simulink model "filter_current"  (R2023b)
settings: Solver=FixedStepDiscrete  StartTime=0.0  StopTime=10.0  FixedStep=FilterCurrent_Ts  RelTol=1e-3  EnableMultiTasking=on
model workspace (MAT data in the model file):
  FilterCurrent_Ts = Simulink.Parameter
  FilterCurrent_Ts.Value = 0.001
  FilterCurrent_Ts.DataType = 'auto'
  FilterCurrent_Ts.DocUnits = 's'
  FilterCurrent_Ts.Complexity = 'real'
  FilterCurrent_Ts.Dimensions = [1 1]
libraries: dspstat3 x1
settings Model: DataDictionary=common.sldd  Creator=ascalzo  LastModifiedBy=mfussi
settings SolverCC: AllowMultiTaskInputOutput=on  AutoInsertRateTranBlk=on  InsertRTBMode=Never (minimum delay)
settings DataIOCC: SaveOutput=off  SignalLogging=off  DSMLogging=off  SaveTime=off  ReturnWorkspaceOutputs=off
settings OptimizationCC: DefaultParameterBehavior=Inlined  UseDivisionForNetSlopeComputation=on  GainParamInheritBuiltInType=on  UseFloatMulNetSlope=on  DefaultUnderspecifiedDataType=single  InlineInvariantSignals=on  PassReuseOutputArgsAs=Individual arguments  ZeroExternalMemoryAtStartup=off  ZeroInternalMemoryAtStartup=off  NoFixptDivByZeroProtection=on  EfficientFloat2IntCast=on  LifeSpan=1  OptimizeBlockOrder=speed  OptimizationPriority=Speed  MultiThreadedLoops=on  EfficientTunableParamExpr=on
settings DebuggingCC: ParameterPrecisionLossMsg=none  UnconnectedInputMsg=warning  UnconnectedOutputMsg=warning  UnconnectedLineMsg=warning
settings HardwareCC: ProdBitPerPointer=32  ProdBitPerSizeT=32  ProdBitPerPtrDiffT=32  ProdLargestAtomicInteger=Long  ProdLargestAtomicFloat=Double  ProdWordSize=32  ProdLongLongMode=on  ProdHWDeviceType=ARM Compatible->ARM Cortex-M
settings ModelReferenceCC: UpdateModelReferenceTargets=Force  EnableRefExpFcnMdlSchedulingChecks=on
settings SFSimCC: MATLABDynamicMemAlloc=off
settings RTWCC: Description=Embedded Coder  SystemTargetFile=ert.tlc  GenCodeOnly=on  PackageGeneratedCodeAndArtifacts=on  PackageName=filter_current  TemplateMakefile=ert_default_tmf  DLArmComputeVersion=19.05
settings CodeAppCC: ForceParamTrailComments=on  IgnoreCustomStorageClasses=off  MaxIdLength=60  OperatorAnnotations=on  SimulinkDataObjDesc=on  SFDataObjDesc=on  InsertBlockDesc=on
settings ERTTargetCC: TargetLangStandard=C99 (ISO)  CodeReplacementLibrary=ARM Cortex-M,iCubTech  GenerateSampleERTMain=on  IncludeMdlTerminateFcn=off  CombineSignalStateStructs=on  SuppressErrorStatus=on  SupportAbsoluteTime=off  CodeInterfacePackaging=Reusable function  SupportComplex=off  InlinedParameterPlacement=NonHierarchical  RootIOFormat=Structure reference  ERTCustomFileTemplate=example_file_process.tlc  ERTFilePackagingFormat=CompactWithDataFile

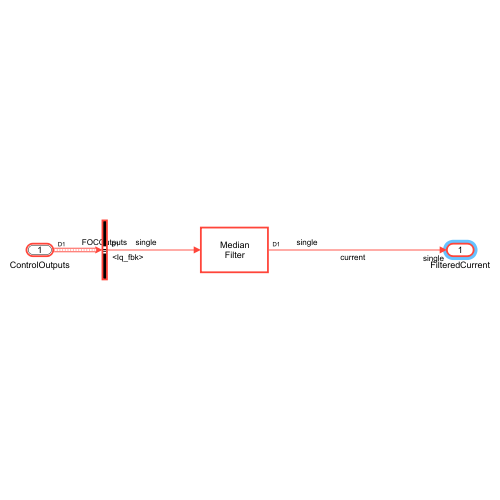
[thumbnail: Simulink's stored preview of the top-level diagram]
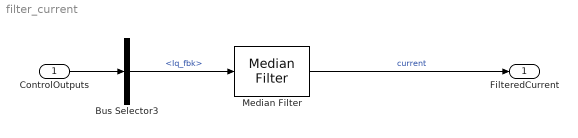
== system filter_current ==
  ControlOutputs : Inport  OutDataTypeStr=Bus: FOCOutputs  BusOutputAsStruct=on
  Bus Selector3 : BusSelector  OutputSignals=Iq_fbk
  Median Filter : dspstat3/Median Filter  WindowLength=32  SimulateUsing=Code generation
  FilteredCurrent : Outport  OutDataTypeStr=single  Unit=A  BusOutputAsStruct=on
  wires:
  ControlOutputs/1 -> Bus Selector3/1
  Bus Selector3/1 -> Median Filter/1  "<Iq_fbk>"
  Median Filter/1 -> FilteredCurrent/1  "current"
